simulink model "lab4b"  (R2024b)
settings: Solver=VariableStepAuto  StartTime=0.0  StopTime=10.0  RelTol=1e-3
undefined symbols (not defined in the file or in its folder): Angle, Magnitude
libraries: spsVoltageMeasurementLib x3, spsCurrentMeasurementLib x3, spsLinearTransformerLib x2, spsSeriesRLCBranchLib x2, spsACVoltageSourceLib x1, sps_lib x1
settings Model: Creator=Jamil!  LastModifiedBy=Jamil!

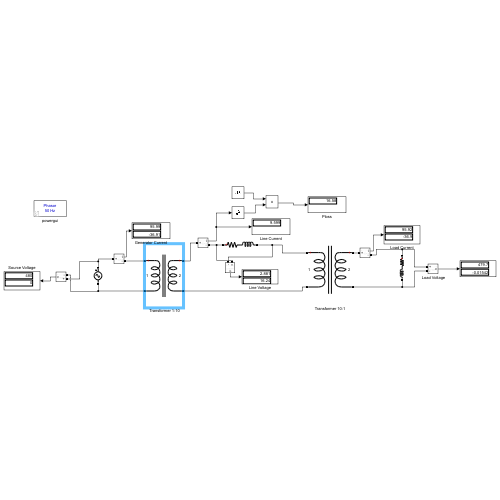
[thumbnail: Simulink's stored preview of the top-level diagram]
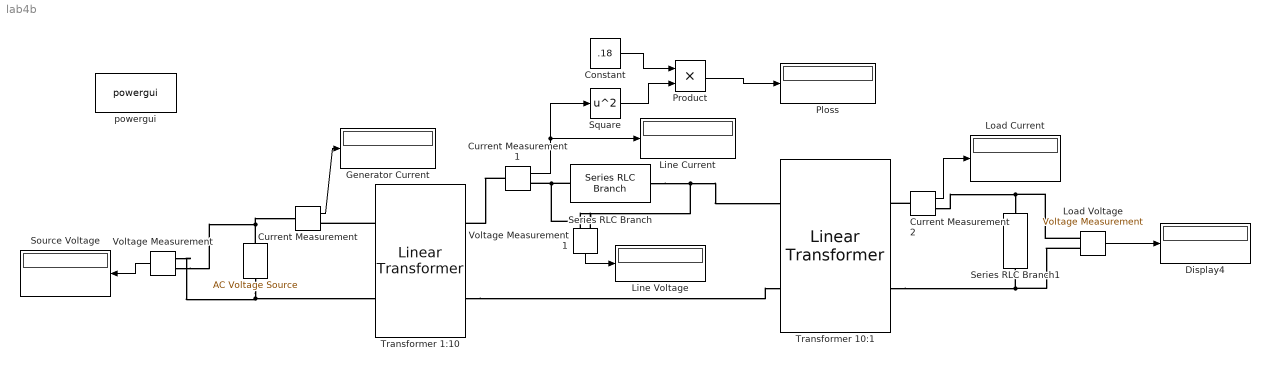
== system lab4b ==
  " " : spsACVoltageSourceLib/AC Voltage Source  Amplitude=480  Phase=0  Frequency=50  SampleTime=0  Measurements=None  BusType=swing  Pref=10e3  Qref=0  Qmin=-inf  Qmax=+inf
  " Load Voltage" : spsVoltageMeasurementLib/Voltage Measurement  PhasorSimulation=on  OutputType=Magnitude-Angle  PSBequivalent=0
  " Transformer 1:10" : spsLinearTransformerLib/Linear Transformer  UNITS=SI  NominalPower=[ 250e6 60 ]  winding1=[480 .000001 .000001]  winding2=[4800 .000001 .000001]  ThreeWindings=off  winding3=[3.15e+05 0.7938 0.084225]  RmLm=[1.0804e+06 2866]  Measurements=None  DataType=on
  Constant : Constant  Value=.18
  Current Measurement : spsCurrentMeasurementLib/Current Measurement  PhasorSimulation=on  OutputType=Magnitude-Angle  PSBequivalent=0
  Current Measurement1 : spsCurrentMeasurementLib/Current Measurement  PhasorSimulation=on  OutputType=Magnitude  PSBequivalent=0
  Current Measurement2 : spsCurrentMeasurementLib/Current Measurement  PhasorSimulation=on  OutputType=Magnitude-Angle  PSBequivalent=0
  Display4 : Display
      settings: Decimation=2
  Generator Current : Display
      settings: Decimation=2
  Line Current : Display
  Line Voltage : Display
      settings: Decimation=2
  Load Current : Display
      settings: Decimation=2
  Ploss : Display
      settings: Decimation=2
  Product : Product
  Series RLC Branch : spsSeriesRLCBranchLib/Series RLC Branch  LConnTagsString=__new0  RConnTagsString=__new0  BranchType=RL  Resistance=.18  Inductance=0.0007643312  SetiL0=off  InitialCurrent=0  Capacitance=1e-6  Setx0=off  InitialVoltage=0  Measurements=None
  Series RLC Branch1 : spsSeriesRLCBranchLib/Series RLC Branch  LConnTagsString=__new0  RConnTagsString=__new0  BranchType=RL  Resistance=4  Inductance=0.0095541401  SetiL0=off  InitialCurrent=0  Capacitance=1e-6  Setx0=off  InitialVoltage=0  Measurements=None
  Source Voltage : Display
  Square : Math  Operator=square
  Transformer 10:1 : spsLinearTransformerLib/Linear Transformer  UNITS=SI  NominalPower=[ 250e6 60 ]  winding1=[4800 .000001 .000001]  winding2=[480 .000001 .000001]  ThreeWindings=off  winding3=[3.15e+05 0.7938 0.084225]  RmLm=[1.0804e+06 2866]  Measurements=None  DataType=on
  Voltage Measurement : spsVoltageMeasurementLib/Voltage Measurement  PhasorSimulation=on  OutputType=Magnitude-Angle  PSBequivalent=0
  Voltage Measurement1 : spsVoltageMeasurementLib/Voltage Measurement  PhasorSimulation=on  OutputType=Magnitude-Angle  PSBequivalent=0
  powergui : sps_lib/powergui  Priority=1  SimulationMode=Phasor  SampleTime=50e-6  frequency=50  Iterations=50  frequencyindice=50  Pbase=100e6  ErrMax=1e-4  UnitsV=kV  UnitsW=MW  buscounter=0  FunctionMessages=off  echomessages=off  EnableUseOfTLC=off  CurrentSourceSwitches=off  DisableSnubberDevices=off  DisableRonSwitches=off  DisableVfSwitches=off  DisplayEquations=off  AutomaticDiscreteSolvers=off  SolverType=Tustin/Backward Euler (TBE)  Interpol=off  ExternalGateDelay=off  methode=off  Ts=100  x0status=blocks  SPID=on  SwTol=0  HookPort=off  NonlinearTolerance=1e-4  nMaxIteration=100  ContinueOnMaxIteration=off  RestoreLinks=warning  ResistiveCurrentMeasurement=off  Frange=[0:2:500]  Ylog=off  Xlog=on  ShowGrid=off  save=off  variable=ZData  structure=0  ZoomFFT=off  StartTime=0.0  cycles=1  DisplayStyle=1  fundamental=60  FreqAxis=off  MaxFrequency=1000  frequencyindicesteady=1  RmsSteady=1  display=off
  wires:
  Square/1 -> Product/2
  Constant/1 -> Product/1
  Product/1 -> Ploss/1
  Current Measurement1/1 -> Square/1, Line Current/1
  Voltage Measurement1/1 -> Line Voltage/1
  " Load Voltage"/1 -> Display4/1
  Voltage Measurement/1 -> Source Voltage/1
  Current Measurement/1 -> Generator Current/1
  Current Measurement2/1 -> Load Current/1
  connections:
  " "/RConn1 -- Voltage Measurement/LConn1 -- Current Measurement/LConn1
  " Transformer 1:10"/LConn1 -- Current Measurement/RConn1
  " "/LConn1 -- Voltage Measurement/LConn2 -- " Transformer 1:10"/LConn2
  Current Measurement1/LConn1 -- " Transformer 1:10"/RConn1
  Series RLC Branch/LConn1 -- Voltage Measurement1/LConn1 -- Current Measurement1/RConn1
  Series RLC Branch/RConn1 -- Voltage Measurement1/LConn2 -- Transformer 10:1/LConn1
  " Transformer 1:10"/RConn2 -- Transformer 10:1/LConn2
  Current Measurement2/LConn1 -- Transformer 10:1/RConn1
  Current Measurement2/RConn1 -- Series RLC Branch1/LConn1 -- " Load Voltage"/LConn1
  Transformer 10:1/RConn2 -- Series RLC Branch1/RConn1 -- " Load Voltage"/LConn2
